simulink model "heli_q8_lab2_DELETE_ME"  (R2019b)
settings: Solver=ode1  StartTime=0.0  StopTime=inf  FixedStep=0.002  RelTol=1e-3  EnableMultiTasking=on
PostLoadFcn:
  | qc_set_target_type(getConfigSet(bdroot, 'QUARC Default Target Configuration'));
values from neighbouring files (symbols this model uses):
  F = [k_11 k_13; k_21 k_23]    [lab2.m]
  K = lqr(A_a, B_a, Q, R)    [lab2.m]
  K1 = l_p*Kf/(2*m_p*l_p^2)    [PDcontrol.m]
  pole1 = -5 + 3i    [PDcontrol.m]
  pole2 = conj(pole1)    [PDcontrol.m]
  Vs0 = 5.48    [PDcontrol.m]
undefined symbols (not defined in the file or in its folder): HIL, Joystick_gain_x, Joystick_gain_y, qc_get_step_size
libraries: quarc_library x4
settings Model: SimulationMode=external  ExtModeTrigDuration=30000  Creator=Rchan  LastModifiedBy=andre
settings SolverCC: PositivePriorityOrder=on
settings DataIOCC: LimitDataPoints=on  SaveFormat=Array  SignalLoggingSaveFormat=ModelDataLogs  ReturnWorkspaceOutputs=off
settings OptimizationCC: ExpressionDepthLimit=2147483647  InitFltsAndDblsToZero=on  LifeSpan=inf
settings DebuggingCC: SaveWithParameterizedLinksMsg=none  UnderspecifiedInitializationDetection=Classic  MergeDetectMultiDrivingBlocksExec=none  SolverPrmCheckMsg=warning  MultiTaskDSMMsg=warning  MultiTaskCondExecSysMsg=none  FcnCallInpInsideContextMsg=warning  AllowSymbolicDim=off  StateNameClashWarn=warning  SFUnexpectedBacktrackingDiag=warning  SFNoUnconditionalDefaultTransitionDiag=warning  SFExecutionAtInitializationDiag=none  ArithmeticOperatorsInVariantConditions=warning
settings HardwareCC: ProdBitPerPointer=32  ProdBitPerSizeT=32  ProdBitPerPtrDiffT=32  ProdLargestAtomicFloat=None  ProdIntDivRoundTo=Undefined  ProdEndianess=Unspecified  ProdWordSize=32  ProdHWDeviceType=32-bit Generic
settings ModelReferenceCC: PropagateSignalLabelsOutOfModel=off
settings SFSimCC: SimUseLocalCustomCode=off  CustomCodeUndefinedFunction=UseInterfaceOnly
settings RTWCC: Description=QUARC Win64 Target  SystemTargetFile=quarc_win64.tlc  TemplateMakefile=quarc_default_tmf  RTWUseLocalCustomCode=off
settings CodeAppCC: StateflowObjectComments=on
settings STFCustomTargetCC: TargetPreCompLibLocation=C:\PROGRA~3\QUARC\lib\2015b\win64\release  ConcurrentExecutionCompliant=on  GeneratePreprocessorConditionals=Disable all  CPPClassGenCompliant=on  GRTInterface=on  SystemTargetFile=quarc_win64.tlc
settings GRTTargetCC: TargetPreCompLibLocation=C:\PROGRA~3\QUARC\lib\2015b\win64\release  TargetLangStandard=C89/C90 (ANSI)  ParMdlRefBuildCompliant=off  CompOptLevelCompliant=off  GeneratePreprocessorConditionals=Disable all  CombineOutputUpdateFcns=off  MatFileLogging=off  GRTInterface=on  UseToolchainInfoCompliant=off  ExtMode=on  ExtModeMexFile=quarc_comm
settings ConfigComp: CovMetricSettings=dw  CovHtmlReporting=on  CovSaveCumulativeToWorkspaceVar=on  CovSaveSingleToWorkspaceVar=on  CovExternalEMLEnable=off  CovSFcnEnable=off

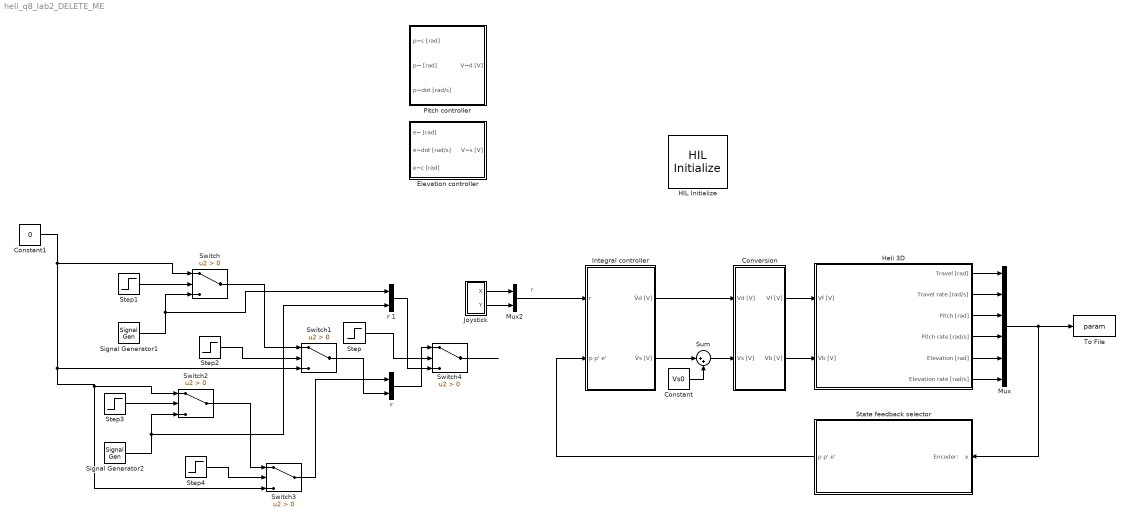
== system heli_q8_lab2_DELETE_ME ==
  note: r
  Constant : Constant  Value=Vs0
  Constant1 : Constant  Value=0
  Conversion : Subsystem
  Elevation controller : Subsystem
  HIL Initialize : quarc_library/Data Acquisition/Generic/Configuration/HIL Initialize  Priority=-99  object_name=HIL-1  board_type=q8_usb  board_number=0  board_options=update_rate=normal;decimation=1  exclusive=off  active=off  hardware_clocks=[0:2]  clock_modes=[]  initial_clock_frequencies=[]  set_clock_params_at_start=off  set_clock_params_at_switch_in=off  set_clock_frequencies_at_start=off  set_clock_frequencies_at_switch_in=off  analog_input_channels=[0:7]  analog_input_maximums=10  analog_input_minimums=-10  set_analog_input_params_at_start=on  set_analog_input_params_at_switch_in=off  analog_output_channels=[0:7]  analog_output_maximums=10  analog_output_minimums=-10  initial_analog_outputs=[0]  final_analog_outputs=[0]  watchdog_analog_outputs=0  set_analog_output_params_at_start=on  set_analog_output_params_at_switch_in=off  set_analog_outputs_at_start=on  set_analog_outputs_at_switch_in=off  set_analog_outputs_at_terminate=on  set_analog_outputs_at_switch_out=off  set_analog_outputs_on_watchdog=off  digital_input_channels=[]  digital_output_channels=[]  digital_output_configuration=[]  initial_digital_outputs=[1]  final_digital_outputs=[1]  watchdog_digital_outputs=[1]  set_digital_output_params_at_start=off  set_digital_output_params_at_switch_in=off  set_digital_outputs_at_start=on  set_digital_outputs_at_switch_in=off  set_digital_outputs_at_terminate=on  set_digital_outputs_at_switch_out=off  set_digital_outputs_on_watchdog=off  encoder_channels=[0:7]  quadrature=[4]  encoder_filter_frequency=[]  initial_encoder_counts=[0]  set_encoder_params_at_start=on  set_encoder_params_at_switch_in=off  set_encoder_counts_at_start=on  set_encoder_counts_at_switch_in=off  pwm_channels=[0:7]  pwm_modes=0  pwm_frequency=99.532799999999995e6/4095  pwm_configuration=[0]  pwm_alignment=[0]  pwm_polarity=[1]  pwm_leading_deadband=[0]  pwm_trailing_deadband=[0]  initial_pwm_outputs=[0]  final_pwm_outputs=[0]  watchdog_pwm_outputs=[0]  set_pwm_params_at_start=on  set_pwm_params_at_switch_in=off  set_pwm_outputs_at_start=on  set_pwm_outputs_at_switch_in=off  set_pwm_outputs_at_terminate=on  set_pwm_outputs_at_switch_out=off  set_pwm_outputs_on_watchdog=off  other_output_channels=[]  initial_other_outputs=[]  final_other_outputs=[]  watchdog_other_outputs=[]  set_other_outputs_at_start=off  set_other_outputs_at_switch_in=off  set_other_outputs_at_terminate=off  set_other_outputs_at_switch_out=off  set_other_outputs_on_watchdog=off
  Heli 3D : Subsystem
  Integral controller : Subsystem
  Joystick : Subsystem
  Mux : Mux  Inputs=6
  Mux2 : Mux  Inputs=2
  Pitch controller : Subsystem
  Signal Generator1 : SignalGenerator  Units=rad/sec
  Signal Generator2 : SignalGenerator  Units=rad/sec
  State feedback selector : Subsystem
  Step : Step  Time=30  SampleTime=0
  Step1 : Step  Time=5  SampleTime=0
  Step2 : Step  Time=10  SampleTime=0
  Step3 : Step  Time=15  SampleTime=0
  Step4 : Step  Time=20  SampleTime=0
  Sum : Sum  Inputs=|++
  Switch{,1..4} (5 alike) : Switch  Criteria=u2 > Threshold
  To File : ToFile  Filename=param
  "r " : Concatenate
  r 1 : Concatenate
  wires:
  Conversion/2(Vb [V]) -> Heli 3D/2(Vb [V])
  Conversion/1(Vf [V]) -> Heli 3D/1(Vf [V])
  Heli 3D/1(Travel [rad]) -> Mux/1
  Heli 3D/2(Travel rate [rad/s]) -> Mux/2
  Heli 3D/3(Pitch [rad]) -> Mux/3
  Heli 3D/4(Pitch rate [rad/s]) -> Mux/4
  Heli 3D/5(Elevation [rad]) -> Mux/5
  Heli 3D/6(Elevation rate [rad/s]) -> Mux/6
  Mux/1 -> State feedback selector/1(Encoder:    x), To File/1
  Constant/1 -> Sum/2
  Sum/1 -> Conversion/2(Vs [V])
  State feedback selector/1(p p' e') -> Integral controller/2(p p' e')
  Joystick/1(X) -> Mux2/1
  Joystick/2(Y) -> Mux2/2
  "r "/1 -> Switch4/1
  Integral controller/2(Ṽs [V]) -> Sum/1
  Integral controller/1(Ṽd [V]) -> Conversion/1(Vd [V])
  Step1/1 -> Switch/2
  Constant1/1 -> Switch2/1, Switch3/3, Switch1/3, Switch/1
  Signal Generator1/1 -> r 1/1, Switch/3
  Switch/1 -> Switch1/1
  Step2/1 -> Switch1/2
  Switch1/1 -> "r "/2
  Step3/1 -> Switch2/2
  Switch2/1 -> Switch3/1
  Step4/1 -> Switch3/2
  Switch3/1 -> "r "/1
  Signal Generator2/1 -> r 1/2, Switch2/3
  r 1/1 -> Switch4/3
  Step/1 -> Switch4/2
  Switch4/1 -> ?
  Mux2/1 -> Integral controller/1(r)

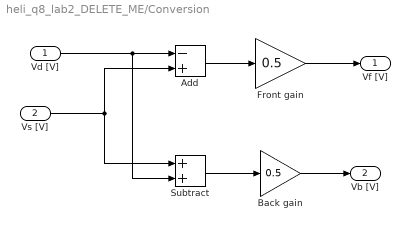
== system heli_q8_lab2_DELETE_ME/Conversion ==
  Vd [V] : Inport
  Vs [V] : Inport  Port=2
  Add : Sum  Inputs=-+
  Back gain : Gain  Gain=0.5
  Front gain : Gain  Gain=0.5
  Subtract : Sum
  Vf [V] : Outport  VectorParamsAs1DForOutWhenUnconnected=off
  Vb [V] : Outport  Port=2  VectorParamsAs1DForOutWhenUnconnected=off
  wires:
  Vd [V]/1 -> Subtract/2, Add/1
  Vs [V]/1 -> Subtract/1, Add/2
  Subtract/1 -> Back gain/1
  Back gain/1 -> Vb [V]/1
  Add/1 -> Front gain/1
  Front gain/1 -> Vf [V]/1

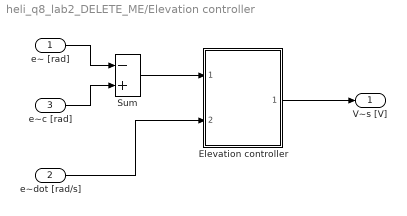
== system heli_q8_lab2_DELETE_ME/Elevation controller ==
  e~ [rad] : Inport
  e~dot [rad/s] : Inport  Port=2
  e~c [rad] : Inport  Port=3
  Elevation controller : Subsystem
  Sum : Sum  Inputs=-+  SaturateOnIntegerOverflow=on  InputSameDT=on  OutDataTypeStr=Inherit: Same as first input
  V~s [V] : Outport  InitialOutput=0  VectorParamsAs1DForOutWhenUnconnected=off
  wires:
  Sum/1 -> Elevation controller/1(e~ [rad])
  Elevation controller/1(V~_s [V]) -> V~s [V]/1
  e~ [rad]/1 -> Sum/1
  e~dot [rad/s]/1 -> Elevation controller/2(e~_dot [rad/s])
  e~c [rad]/1 -> Sum/2

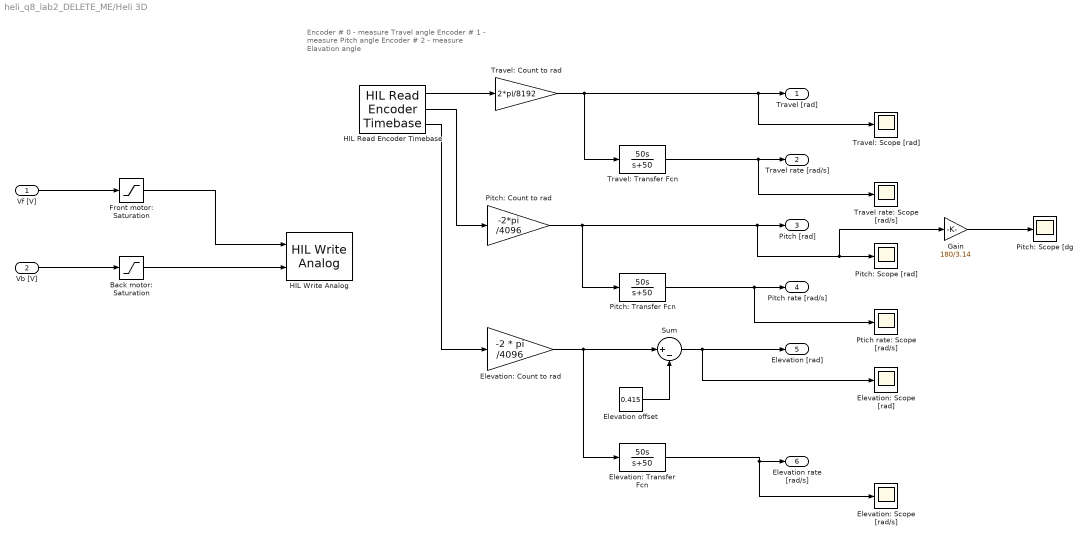
== system heli_q8_lab2_DELETE_ME/Heli 3D ==
  note: Encoder # 0 - measure Travel angle
      | Encoder # 1 - measure Pitch angle
      | Encoder # 2 - measure Elavation angle
  Vf [V] : Inport
  Vb [V] : Inport  Port=2
  Back motor: Saturation : Saturate  UpperLimit=5  LowerLimit=-5
  Elevation offset : Constant  Value=0.415
  Elevation: Count to rad : Gain  Gain=-2 * pi /4096
  Elevation: Scope [rad/s] : Scope
  Elevation: Scope [rad] : Scope
  Elevation: Transfer Fcn : TransferFcn  Numerator=[50 0]  Denominator=[1 50]
  Front motor: Saturation : Saturate  UpperLimit=5  LowerLimit=-5
  Gain : Gain  Gain=180/3.14
  HIL Read Encoder Timebase : quarc_library/Data Acquisition/Generic/Timebases/HIL Read Encoder Timebase  object_name=HIL-1  clock=0  channels=[0:2]  samples_in_buffer=max(ceil(1/qc_get_step_size), 1)  active=on  vector_output=off  data_type_mode=Inherit via back propagation  data_type=double
  HIL Write Analog : quarc_library/Data Acquisition/Generic/Immediate I//O/HIL Write Analog  object_name=HIL-1  channels=[0:1]  sample_time=-1  active=off  vector_input=off
  Pitch: Count to rad : Gain  Gain=-2*pi /4096
  Pitch: Scope [dg : Scope
  Pitch: Scope [rad] : Scope
  Pitch: Transfer Fcn : TransferFcn  Numerator=[50 0]  Denominator=[1 50]
  Ptich rate: Scope [rad/s] : Scope
  Sum : Sum  Inputs=|+-
  Travel rate: Scope [rad/s] : Scope
  Travel: Count to rad : Gain  Gain=2*pi/8192
  Travel: Scope [rad] : Scope
  Travel: Transfer Fcn : TransferFcn  Numerator=[50 0]  Denominator=[1 50]
  Travel [rad] : Outport  VectorParamsAs1DForOutWhenUnconnected=off
  Travel rate [rad/s] : Outport  Port=2  VectorParamsAs1DForOutWhenUnconnected=off
  Pitch [rad] : Outport  Port=3  VectorParamsAs1DForOutWhenUnconnected=off
  Pitch rate [rad/s] : Outport  Port=4  VectorParamsAs1DForOutWhenUnconnected=off
  Elevation [rad] : Outport  Port=5  VectorParamsAs1DForOutWhenUnconnected=off
  Elevation rate [rad/s] : Outport  Port=6  VectorParamsAs1DForOutWhenUnconnected=off
  wires:
  HIL Read Encoder Timebase/1 -> Travel: Count to rad/1
  HIL Read Encoder Timebase/2 -> Pitch: Count to rad/1
  HIL Read Encoder Timebase/3 -> Elevation: Count to rad/1
  Travel: Count to rad/1 -> Travel: Scope [rad]/1, Travel [rad]/1, Travel: Transfer Fcn/1
  Travel: Transfer Fcn/1 -> Travel rate: Scope [rad/s]/1, Travel rate [rad/s]/1
  Pitch: Count to rad/1 -> Pitch: Transfer Fcn/1, Gain/1, Pitch: Scope [rad]/1, Pitch [rad]/1
  Pitch: Transfer Fcn/1 -> Ptich rate: Scope [rad/s]/1, Pitch rate [rad/s]/1
  Elevation: Count to rad/1 -> Sum/1, Elevation: Transfer Fcn/1
  Elevation: Transfer Fcn/1 -> Elevation: Scope [rad/s]/1, Elevation rate [rad/s]/1
  Vf [V]/1 -> Front motor: Saturation/1
  Vb [V]/1 -> Back motor: Saturation/1
  Front motor: Saturation/1 -> HIL Write Analog/1
  Back motor: Saturation/1 -> HIL Write Analog/2
  Elevation offset/1 -> Sum/2
  Sum/1 -> Elevation: Scope [rad]/1, Elevation [rad]/1
  Gain/1 -> Pitch: Scope [dg/1

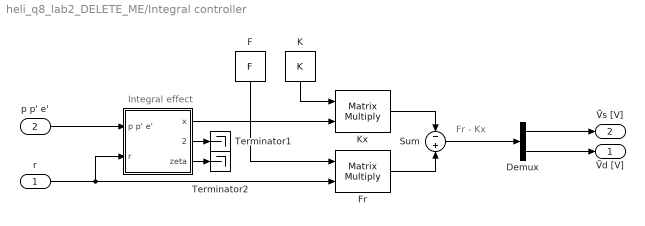
== system heli_q8_lab2_DELETE_ME/Integral controller ==
  note: Integral effect
  note: Fr - Kx
  r : Inport
  p p' e' : Inport  Port=2
  "                         " : Subsystem
  Demux : Demux  Outputs=2
  F : Constant  Value=F  VectorParams1D=off
  Fr : Product  Multiplication=Matrix(*)
  K : Constant  Value=K  VectorParams1D=off
  Kx : Product  Multiplication=Matrix(*)  RndMeth=Nearest  OutDataTypeStr=Inherit: Same as first input
  Sum : Sum  Inputs=-|+
  Terminator1 : Terminator
  Terminator2 : Terminator
  Ṽd [V] : Outport  InitialOutput=0
  Ṽs [V] : Outport  Port=2  InitialOutput=0
  wires:
  K/1 -> Kx/1
  p p' e'/1 -> "                         "/1(p p' e')
  F/1 -> Fr/1
  Fr/1 -> Sum/2
  Kx/1 -> Sum/1
  Sum/1 -> Demux/1
  Demux/1 -> Ṽs [V]/1
  Demux/2 -> Ṽd [V]/1
  r/1 -> Fr/2, "                         "/2(r)
  "                         "/1(x) -> Kx/2
  "                         "/2(gamma) -> Terminator1/1
  "                         "/3(zeta) -> Terminator2/1

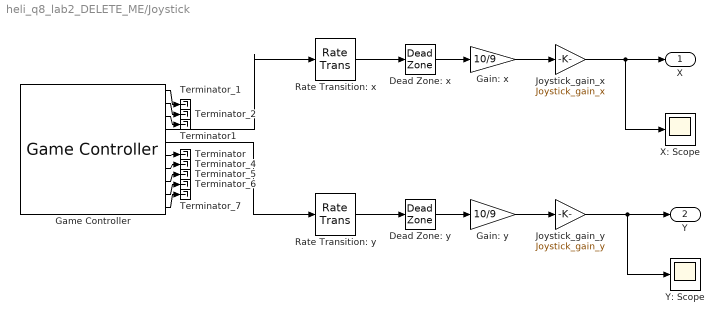
== system heli_q8_lab2_DELETE_ME/Joystick ==
  Dead Zone: x : DeadZone  LowerValue=-0.1  UpperValue=0.1  SaturateOnIntegerOverflow=on
  Dead Zone: y : DeadZone  LowerValue=-0.1  UpperValue=0.1  SaturateOnIntegerOverflow=on
  Gain: x : Gain  Gain=10/9
  Gain: y : Gain  Gain=10/9
  Game Controller : quarc_library/Devices/Peripherals/Target/Game Controller  controller=1  buffer_size=12  deadzone=[]  saturation=[]  sample_time=max(qc_get_step_size, 0.01)  auto_center=off  enabled=on
  Joystick_gain_x : Gain  Gain=Joystick_gain_x
  Joystick_gain_y : Gain  Gain=Joystick_gain_y
  Rate Transition: x : RateTransition
  Rate Transition: y : RateTransition
  Terminator : Terminator
  Terminator1 : Terminator
  Terminator_{1..2,4..7} (6 alike) : Terminator
  X: Scope : Scope
  Y: Scope : Scope
  X : Outport  VectorParamsAs1DForOutWhenUnconnected=off
  Y : Outport  Port=2  VectorParamsAs1DForOutWhenUnconnected=off
  wires:
  Rate Transition: y/1 -> Dead Zone: y/1
  Rate Transition: x/1 -> Dead Zone: x/1
  Game Controller/5 -> Rate Transition: y/1
  Game Controller/4 -> Rate Transition: x/1
  Game Controller/1 -> Terminator_1/1
  Game Controller/2 -> Terminator_2/1
  Game Controller/7 -> Terminator_4/1
  Game Controller/8 -> Terminator_5/1
  Game Controller/9 -> Terminator_6/1
  Game Controller/10 -> Terminator_7/1
  Game Controller/3 -> Terminator1/1
  Game Controller/6 -> Terminator/1
  Dead Zone: x/1 -> Gain: x/1
  Dead Zone: y/1 -> Gain: y/1
  Gain: x/1 -> Joystick_gain_x/1
  Gain: y/1 -> Joystick_gain_y/1
  Joystick_gain_x/1 -> X/1, X: Scope/1
  Joystick_gain_y/1 -> Y: Scope/1, Y/1

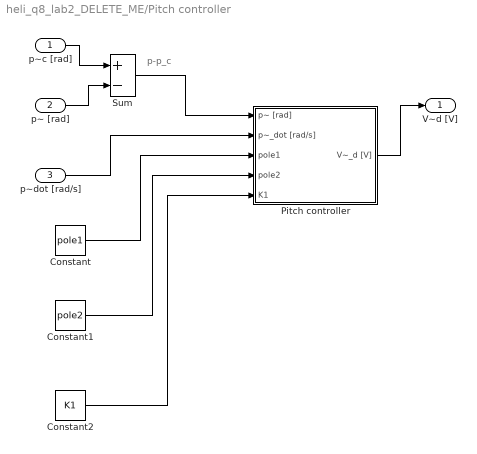
== system heli_q8_lab2_DELETE_ME/Pitch controller ==
  note: p-p_c
  p~c [rad] : Inport
  p~ [rad] : Inport  Port=2
  p~dot [rad/s] : Inport  Port=3
  Constant : Constant  Value=pole1
  Constant1 : Constant  Value=pole2
  Constant2 : Constant  Value=K1
  Pitch controller : Subsystem
  Sum : Sum  Inputs=+-  SaturateOnIntegerOverflow=on  InputSameDT=on  OutDataTypeStr=Inherit: Same as first input
  V~d [V] : Outport  InitialOutput=0  VectorParamsAs1DForOutWhenUnconnected=off
  wires:
  Sum/1 -> Pitch controller/1(p~ [rad])
  Pitch controller/1(V~_d [V]) -> V~d [V]/1
  p~c [rad]/1 -> Sum/1
  p~dot [rad/s]/1 -> Pitch controller/2(p~_dot [rad/s])
  p~ [rad]/1 -> Sum/2
  Constant/1 -> Pitch controller/3(pole1)
  Constant1/1 -> Pitch controller/4(pole2)
  Constant2/1 -> Pitch controller/5(K1)

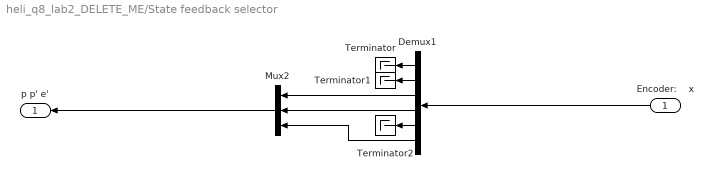
== system heli_q8_lab2_DELETE_ME/State feedback selector ==
  Encoder:    x : Inport
  Demux1 : Demux  Outputs=6
  Mux2 : Mux  Inputs=3
  Terminator : Terminator
  Terminator1 : Terminator
  Terminator2 : Terminator
  p p' e' : Outport
  wires:
  Encoder:    x/1 -> Demux1/1
  Demux1/3 -> Mux2/1
  Demux1/4 -> Mux2/2
  Demux1/6 -> Mux2/3
  Mux2/1 -> p p' e'/1
  Demux1/1 -> Terminator/1
  Demux1/2 -> Terminator1/1
  Demux1/5 -> Terminator2/1

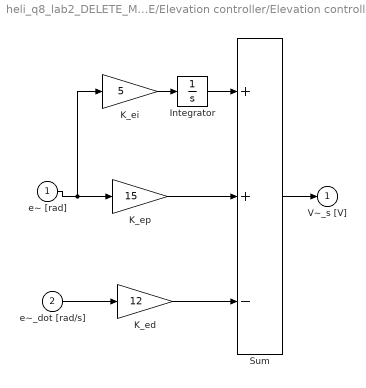
== system heli_q8_lab2_DELETE_ME/Elevation controller/Elevation controller ==
  e~ [rad] : Inport
  e~_dot [rad/s] : Inport  Port=2
  Integrator : Integrator  LimitOutput=on
  K_ed : Gain  Gain=12  SaturateOnIntegerOverflow=on  OutDataTypeStr=Inherit: Same as input  ParamDataTypeStr=Inherit: Same as input
  K_ei : Gain  Gain=5  SaturateOnIntegerOverflow=on  OutDataTypeStr=Inherit: Same as input  ParamDataTypeStr=Inherit: Same as input
  K_ep : Gain  Gain=15  SaturateOnIntegerOverflow=on  OutDataTypeStr=Inherit: Same as input  ParamDataTypeStr=Inherit: Same as input
  Sum : Sum  Inputs=++-  SaturateOnIntegerOverflow=on  InputSameDT=on  OutDataTypeStr=Inherit: Same as first input
  V~_s [V] : Outport  InitialOutput=0  VectorParamsAs1DForOutWhenUnconnected=off
  wires:
  K_ei/1 -> Integrator/1
  Integrator/1 -> Sum/1
  Sum/1 -> V~_s [V]/1
  e~_dot [rad/s]/1 -> K_ed/1
  K_ed/1 -> Sum/3
  K_ep/1 -> Sum/2
  e~ [rad]/1 -> K_ep/1, K_ei/1

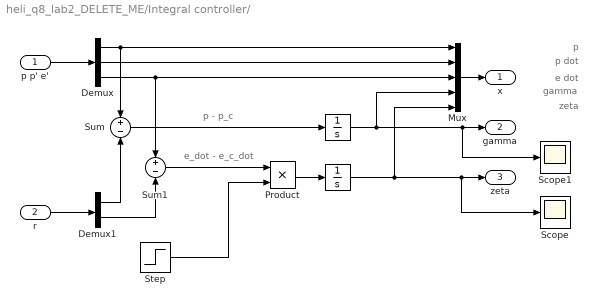
== system heli_q8_lab2_DELETE_ME/Integral controller/                          ==
  note: e dot
  note: p dot
  note: p
  note: gamma
  note: zeta
  note: e_dot - e_c_dot
  note: p - p_c
  p p' e' : Inport
  r : Inport  Port=2
  "  " : Integrator
  "   " : Integrator
  Demux : Demux  Outputs=3
  Demux1 : Demux  Outputs=2
  Mux : Mux  Inputs=5
  Product : Product
  Scope : Scope
  Scope1 : Scope
  Step : Step  Time=5  SampleTime=0
  Sum : Sum  Inputs=+|-
  Sum1 : Sum  Inputs=+|-
  x : Outport
  gamma : Outport  Port=2
  zeta : Outport  Port=3
  wires:
  p p' e'/1 -> Demux/1
  r/1 -> Demux1/1
  Demux/1 -> Mux/1, Sum/1
  Demux/2 -> Mux/2
  Demux/3 -> Mux/3, Sum1/1
  Mux/1 -> x/1
  Demux1/1 -> Sum/2
  Sum/1 -> "  "/1
  "  "/1 -> Scope1/1, gamma/1, Mux/4
  Demux1/2 -> Sum1/2
  Sum1/1 -> Product/1
  "   "/1 -> zeta/1, Scope/1, Mux/5
  Step/1 -> Product/2
  Product/1 -> "   "/1

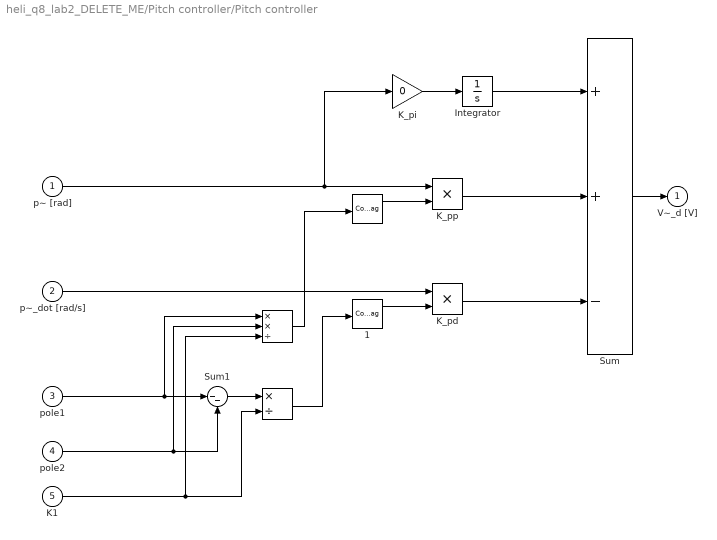
== system heli_q8_lab2_DELETE_ME/Pitch controller/Pitch controller ==
  p~ [rad] : Inport
  p~_dot [rad/s] : Inport  Port=2
  pole1 : Inport  Port=3
  pole2 : Inport  Port=4
  K1 : Inport  Port=5
  " " : Product  Inputs=*/
  "  " : Product  Inputs=**/
  "   " : ComplexToRealImag
  "   1" : ComplexToRealImag
  Integrator : Integrator  LimitOutput=on
  K_pd : Product
  K_pi : Gain  Gain=0  SaturateOnIntegerOverflow=on  OutDataTypeStr=Inherit: Same as input  ParamDataTypeStr=Inherit: Same as input
  K_pp : Product
  Sum : Sum  Inputs=++-  SaturateOnIntegerOverflow=on  InputSameDT=on  OutDataTypeStr=Inherit: Same as first input
  Sum1 : Sum  Inputs=|--
  V~_d [V] : Outport  InitialOutput=0  VectorParamsAs1DForOutWhenUnconnected=off
  wires:
  K_pi/1 -> Integrator/1
  Integrator/1 -> Sum/1
  Sum/1 -> V~_d [V]/1
  p~_dot [rad/s]/1 -> K_pd/1
  K_pd/1 -> Sum/3
  K_pp/1 -> Sum/2
  p~ [rad]/1 -> K_pp/1, K_pi/1
  pole1/1 -> "  "/1, Sum1/1
  pole2/1 -> "  "/2, Sum1/2
  K1/1 -> "  "/3, " "/2
  Sum1/1 -> " "/1
  " "/1 -> "   1"/1
  "  "/1 -> "   "/1
  "   "/1 -> K_pp/2
  "   1"/1 -> K_pd/2
